simulink model "mytest"  (R2018a)
settings: Solver=VariableStepAuto  StartTime=0.0  StopTime=10.0  RelTol=1e-3
undefined symbols (not defined in the file): sigbuilder_block
settings Model: Creator=86188  LastModifiedBy=86188

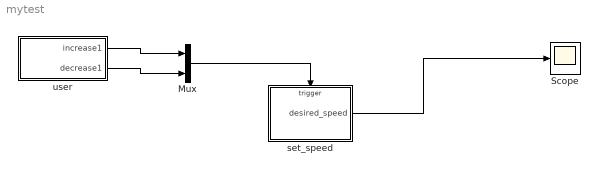
== system mytest ==
  Mux : Mux  Inputs=2
  Scope : Scope
  set_speed : Stateflow chart  TreatAsAtomicUnit=on
  user : Subsystem  Tag=STV Subsys  LoadFcn=sigbuilder_block('load',[4.875 4.875 950.25 537.75 ]);  StartFcn=sigbuilder_block('start');  StopFcn=sigbuilder_block('stop');  ClipboardFcn=sigbuilder_block('clipboard');  mask(Sigbuilder block){tuvar=[0:10]}
      mask help: Simulink:masks:SigbuilderBlock_MD
      mask init:
      | if ~strcmp(get_param(bdroot(gcbh),'SimulationStatus'),'stopped') tuvar = sigbuilder_block('maskInit'); end
      settings: CopyFcn=sigbuilder_block('copy');  DeleteFcn=sigbuilder_block('delete');  ModelCloseFcn=sigbuilder_block('modelClose');  PreSaveFcn=sigbuilder_block('preSave');  PauseFcn=sigbuilder_block('pause');  ContinueFcn=sigbuilder_block('continue');  NameChangeFcn=sigbuilder_block('namechange');  OpenFcn=sigbuilder_block('open',[0 68 1280 636 ]);  CloseFcn=sigbuilder_block('close');
      mask Display: plot(0, 0, 100, 100,[2, 2, 32, 32, 2], [68, 8, 8, 68, 68],[32, 2], [38, 38], [32, 19, 2],[53, 60, 44], [32, 17, 17, 2],[16, 16, 31, 31]);txt = getActiveGroup(gcbh);text(2, 100, txt,'verticalAlignment', 'top');
  wires:
  set_speed/1(desired_speed) -> Scope/1
  user/1(increase1) -> Mux/1
  user/2(decrease1) -> Mux/2
  Mux/1 -> set_speed/Trigger

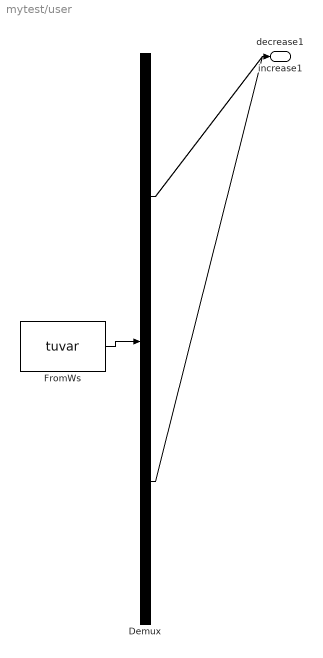
== system mytest/user ==
  Demux : Demux  Tag=STV Demux  Outputs=2
  FromWs : FromWorkspace  Tag=STV FromWs  VariableName=tuvar  SampleTime=0
      SigBuilderData=|
      | common.afterFinalStr = 'Extrapolate'
      | common.sampleTime = 0
      | dataSet.timeRange = [0 10]
      | dataSet.name = 'Group 1'
      | sbobj.Groups.Name = 'Group 1'
      | sbobj.Groups.Signals(1).Name = 'increase1'
      | sbobj.Groups.Signals(1).XData = [0 0.2 0.2 0.4 0.4 0.6 0.6 0.8 0.8 4 6 10]
      | sbobj.Groups.Signals(1).YData = [0 0 1 1 0 0 1 1 0 0 0 0]
      | sbobj.Groups.Signals(2).Name = 'decrease1'
      | sbobj.Groups.Signals(2).XData = [0 4 6 10]
      | sbobj.Groups.Signals(2).YData = [0 0 0 0]
  increase1 : Outport  Tag=STV Outport
  decrease1 : Outport  Tag=STV Outport  Port=2
  wires:
  FromWs/1 -> Demux/1
  Demux/1 -> increase1/1
  Demux/2 -> decrease1/1

== stateflow chart mytest/set_speed ==
  state update
  (default) -> update : {desired_speed=0}
  update -> update [order 1] : increase/{desired_speed = desired_speed + 1}
  update -> update [order 2] : decrease/{desired_speed = desired_speed - 1}
  data: desired_speed output
  events: decrease input EITHER_EDGE_EVENT; increase input EITHER_EDGE_EVENT
